simulink library "GTPR_Library"  (R2021a)
settings: Solver=VariableStepAuto  StartTime=0.0  StopTime=10.0  RelTol=1e-3
values from neighbouring files (symbols this model uses):
  aA = 0.5    [SimMechanics_GTPR_OpenLoop_CircularMotion_VS_ClosedLoop.m]
  aB = 0.5    [SimMechanics_GTPR_OpenLoop_CircularMotion_VS_ClosedLoop.m]
  aC = 0.5    [SimMechanics_GTPR_OpenLoop_CircularMotion_VS_ClosedLoop.m]
  alphaAB = deg2rad(120)    [SimMechanics_GTPR_OpenLoop_CircularMotion_VS_ClosedLoop.m]
  alphaAC = deg2rad(240)    [SimMechanics_GTPR_OpenLoop_CircularMotion_VS_ClosedLoop.m]
  eA = 0.28    [SimMechanics_GTPR_OpenLoop_CircularMotion_VS_ClosedLoop.m]
  eB = 0.28    [SimMechanics_GTPR_OpenLoop_CircularMotion_VS_ClosedLoop.m]
  eC = 0.28    [SimMechanics_GTPR_OpenLoop_CircularMotion_VS_ClosedLoop.m]
  g = -9.81    [SimMechanics_GTPR_OpenLoop_CircularMotion_VS_ClosedLoop.m]
  ILA = zeros(3)    [SimMechanics_GTPR_OpenLoop_CircularMotion_VS_ClosedLoop.m]
  IlA = zeros(3)    [SimMechanics_GTPR_OpenLoop_CircularMotion_VS_ClosedLoop.m]
  ILB = zeros(3)    [SimMechanics_GTPR_OpenLoop_CircularMotion_VS_ClosedLoop.m]
  IlB = zeros(3)    [SimMechanics_GTPR_OpenLoop_CircularMotion_VS_ClosedLoop.m]
  ILC = zeros(3)    [SimMechanics_GTPR_OpenLoop_CircularMotion_VS_ClosedLoop.m]
  IlC = zeros(3)    [SimMechanics_GTPR_OpenLoop_CircularMotion_VS_ClosedLoop.m]
  LA = 0.57    [SimMechanics_GTPR_OpenLoop_CircularMotion_VS_ClosedLoop.m]
  lA = 0.9    [SimMechanics_GTPR_OpenLoop_CircularMotion_VS_ClosedLoop.m]
  LB = 0.57    [SimMechanics_GTPR_OpenLoop_CircularMotion_VS_ClosedLoop.m]
  lB = 0.9    [SimMechanics_GTPR_OpenLoop_CircularMotion_VS_ClosedLoop.m]
  LC = 0.57    [SimMechanics_GTPR_OpenLoop_CircularMotion_VS_ClosedLoop.m]
  lC = 0.9    [SimMechanics_GTPR_OpenLoop_CircularMotion_VS_ClosedLoop.m]
  m_unaccounted = 1e-16    [SimMechanics_GTPR_OpenLoop_CircularMotion_VS_ClosedLoop.m]
  mLA = density_upperArm*VLA    (= 1.4415197891)    [SimMechanics_GTPR_OpenLoop_CircularMotion_VS_ClosedLoop.m]
  mlA = density_LowerArm*VlA    (= 0.190851753706)    [SimMechanics_GTPR_OpenLoop_CircularMotion_VS_ClosedLoop.m]
  mLB = density_upperArm*VLB    (= 1.4415197891)    [SimMechanics_GTPR_OpenLoop_CircularMotion_VS_ClosedLoop.m]
  mlB = density_LowerArm*VlB    (= 0.190851753706)    [SimMechanics_GTPR_OpenLoop_CircularMotion_VS_ClosedLoop.m]
  mLC = density_upperArm*VLC    (= 1.4415197891)    [SimMechanics_GTPR_OpenLoop_CircularMotion_VS_ClosedLoop.m]
  mlC = density_LowerArm*VlC    (= 0.190851753706)    [SimMechanics_GTPR_OpenLoop_CircularMotion_VS_ClosedLoop.m]
  mTCP = density_workTriangle * VTCP    [SimMechanics_GTPR_OpenLoop_CircularMotion_VS_ClosedLoop.m]
undefined symbols (not defined in the file or in its folder): dq1, dq2, dq3, q1, q2, q3, X, Y, Z
libraries: sm_lib x83, $bdroot x31, nesl_utility x24
(part 8 of 8)

== matlab function GTPR_Library/Other Functions/X1/Rz1 ==
  data: theta input; R output
function R = Rz(theta)

R = [cos(theta), -sin(theta), 0; sin(theta), cos(theta), 0; 0,0,1];

== matlab function GTPR_Library/Other Functions/Rz ==
  data: theta input; R output
function R = Rz(theta)

R = [cos(theta), -sin(theta), 0; sin(theta), cos(theta), 0; 0,0,1];

== matlab function GTPR_Library/Other Functions/X2/Rz ==
  data: theta input; R output
function R = Rz(theta)

R = [cos(theta), -sin(theta), 0; sin(theta), cos(theta), 0; 0,0,1];

== matlab function GTPR_Library/Other Functions/Three Spheres Intersection/If Action Subsystem/Simplified - ThreeSpheresIntersection ==
  data: c1 input; upperIntersection output; c2 input; c3 input; r1 input; r2 input; r3 input; lowerIntersection output
function [upperIntersection, lowerIntersection] = SimplifiedThreeSpheresIntersectionAlgorithm(c1,c2,c3,r1,r2,r3)

    % Simplified Three-speheres intersection algorithm from:
    % The Delta Parallel Robot: Kinematics Solutions
    % Robert L. Williams II, Ph.D., williar4@ohio.edu
    % Mechanical Engineering, Ohio University, October 2016
    % Appendix B.

    x1 = c1(1);
    y1 = c1(2);
    z1 = c1(3);

    x2 = c2(1);
    y2 = c2(2);
%     z2 = c2(3);

    x3 = c3(1);
    y3 = c3(2);
%     z3 = c3(3);

    
    a = 2*(x3-x1);
    b = 2*(y3-y1);
    c = power(r1,2)-power(r3,2)-power(x1,2)-power(y1,2)+power(x3,2)+power(y3,2);
    d = 2*(x3-x2);
    e = 2*(y3-y2);
    f = power(r2,2)-power(r3,2)-power(x2,2)-power(y2,2)+power(x3,2)+power(y3,2);

%     aebd = a.*e-b.*d;
% 
%     x = (c.*e-b.*f)./aebd;
%     y = (a.*f-c.*d)./aebd;

    xy = [a b; d e]\[c;f];

    x = xy(1);
    y = xy(2);
    
    A = 1;
    B = -2*z1;
    C = power(z1,2)-power(r1,2)+power(x-x1,2)+power(y-y1,2);

    z = roots([A,B,C]);

    upperIntersection = [x, y, z(1)]';
    lowerIntersection = [x, y, z(2)]';

== matlab function GTPR_Library/Other Functions/X2v/Rz ==
  data: theta input; R output
function R = Rz(theta)

R = [cos(theta), -sin(theta), 0; sin(theta), cos(theta), 0; 0,0,1];
